simulink model "SWC_HALIN_CDD_type"  (R2021b)
settings: Solver=FixedStepDiscrete  StartTime=0.0  StopTime=10.0  FixedStep=0.005  RelTol=1e-3
undefined symbols (not defined in the file or in its folder): C_TASK_5MS_S, DIDLen_APSFunConfig, DIDLen_AutoLock, DIDLen_AutoWipHSpdEN, DIDLen_DKCKey, DIDLen_DRLDis, DIDLen_DynoMode, DIDLen_FMHTimer, DIDLen_OBDReq, DIDLen_TestGroup, DIDLen_TireSize, DIDLen_TurnLampFLThreCurr, DIDLen_TurnLampFRThreCurr, DIDLen_TurnLampRLThreCurr, DIDLen_TurnLampRRThreCurr, DIDLen_USSConfig, DIDLen_WipRLSCmdCutFilter, DIDLen_WipRLSCmdHoldFilter, DIDLen_XWDMode, DIDNum_APSFunConfig, DIDNum_AutoLock, DIDNum_AutoWipHSpdEN, DIDNum_DKCKey, DIDNum_DRLDis, DIDNum_DynoMode, DIDNum_FMHTimer, DIDNum_OBDReq, DIDNum_TestGroup, DIDNum_TireSize, DIDNum_TurnLampFLThreCurr, DIDNum_TurnLampFRThreCurr, DIDNum_TurnLampRLThreCurr, DIDNum_TurnLampRRThreCurr, DIDNum_USSConfig, DIDNum_WipRLSCmdCutFilter, DIDNum_WipRLSCmdHoldFilter, DIDNum_XWDMode, ENUM_DRIVETRAIN_AWD, ENUM_DRIVETRAIN_FWD, ENUM_DRIVETRAIN_RWD, ENUM_REGENLEVEL_LV1, ENUM_REGENLEVEL_LV2, ENUM_REGENLEVEL_LV3, ENUM_REGENLEVEL_LV4, ENUM_REGENLEVEL_LV5, ENUM_REGENLEVEL_OPD, ENUM_TPMSSTA_FAT, ENUM_TPMSSTA_LOWBATTERY, ENUM_TPMSSTA_TRIGGER, FALSE, FIVE_INT, FOUR_INT, KHAL_CANBusOffDebounce_s, KHAL_DefaultRegenMode_enum, KHAL_DKCDecryptEnable_flg_ovrdflg, KHAL_DKCDecryptEnable_flg_ovrdval, KHAL_RandomNumberY1_enum, KHAL_RandomNumberY2_enum, KHAL_RandomNumberY_ovrdflg, KHAL_TPMSRESBUTT_flg_ovrdflg ... (+9)
libraries: simulink x229, FVT_lib x29, hcu_lib x25, hdlsllib x15
(part 1 of 8)
settings Model: DataDictionary=APPTypes.sldd  Creator=FVT23010  LastModifiedBy=FVT23010
settings DataIOCC: SaveFormat=StructureWithTime
settings OptimizationCC: DefaultParameterBehavior=Inlined  EnhancedBackFolding=on  PassReuseOutputArgsAs=Individual arguments  ZeroExternalMemoryAtStartup=off  ZeroInternalMemoryAtStartup=off  OptimizeBlockOrder=speed  DifferentSizesBufferReuse=on  OptimizationCustomize=off  EfficientTunableParamExpr=on
settings DebuggingCC: ParameterTunabilityLossMsg=error
settings ModelReferenceCC: ModelReferenceNumInstancesAllowed=Single
settings SFSimCC: MATLABDynamicMemAlloc=off
settings RTWCC: Description=AUTOSAR  SystemTargetFile=autosar.tlc  GenCodeOnly=on  TemplateMakefile=ert_default_tmf
settings CodeAppCC: ForceParamTrailComments=on  IgnoreCustomStorageClasses=off  OperatorAnnotations=on  SimulinkDataObjDesc=on  SFDataObjDesc=on  InsertBlockDesc=on
settings STFCustomTargetCC: TargetLangStandard=C99 (ISO)  MultiwordLength=256  ParMdlRefBuildCompliant=on  CompOptLevelCompliant=on  IncludeMdlTerminateFcn=off  CombineOutputUpdateFcns=on  SuppressErrorStatus=on  ERTCustomFileBanners=on  SupportNonFinite=off  SupportComplex=off  SupportContinuousTime=off  SupportNonInlinedSFcns=off  RemoveResetFunc=on  MATLABClassNameForMDSCustomization=Simulink.SoftwareTarget.ERTCustomization  AutosarCompliant=on  GRTInterface=off  UseToolchainInfoCompliant=on  LookupTableObjectStructAxisOrder=2,1,3,4,...  LUTObjectStructOrderEvenSpacing=Size,Table,Breakpoints  SystemTargetFile=autosar.tlc
settings ERTTargetCC: TargetLangStandard=C99 (ISO)  ConcurrentExecutionCompliant=off  IncludeMdlTerminateFcn=off  SuppressErrorStatus=on  SupportNonFinite=off  SupportComplex=off  ModelStepFunctionPrototypeControlCompliant=off  CPPClassGenCompliant=off  AutosarCompliant=on  LookupTableObjectStructAxisOrder=2,1,3,4,...  LUTObjectStructOrderEvenSpacing=Size,Table,Breakpoints  InlinedParameterPlacement=NonHierarchical  ERTCustomFileTemplate=example_file_process.tlc

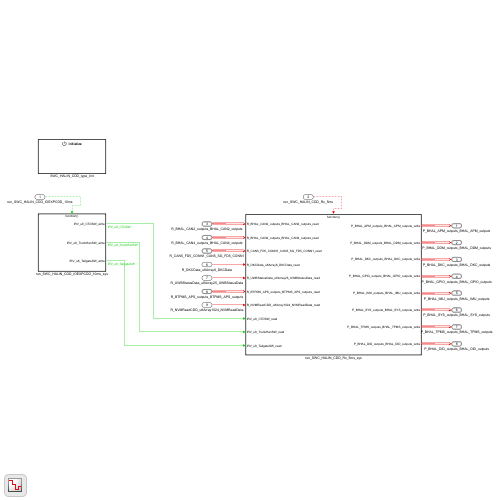
[thumbnail: Simulink's stored preview of the top-level diagram]
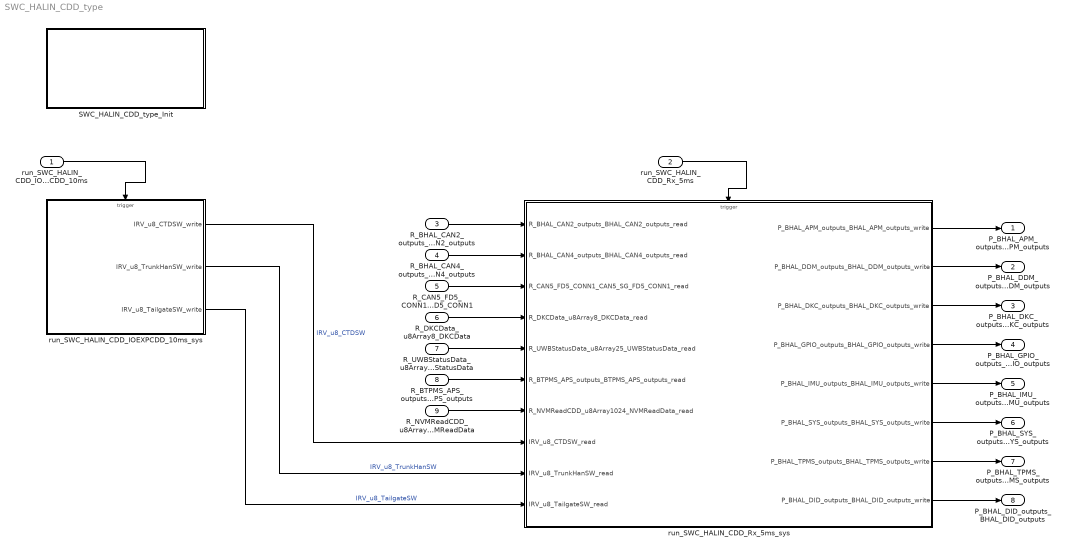
== system SWC_HALIN_CDD_type ==
  run_SWC_HALIN_CDD_IOEXPCDD_10ms : Inport  SampleTime=0.01  OutputFunctionCall=on
  run_SWC_HALIN_CDD_Rx_5ms : Inport  Port=2  SampleTime=0.005  OutputFunctionCall=on
  R_BHAL_CAN2_outputs_BHAL_CAN2_outputs : Inport  Port=3  OutDataTypeStr=Bus: BHAL_CAN2_outputs  PortDimensions=1  BusOutputAsStruct=on
  R_BHAL_CAN4_outputs_BHAL_CAN4_outputs : Inport  Port=4  OutDataTypeStr=Bus: BHAL_CAN4_outputs  PortDimensions=1  BusOutputAsStruct=on
  R_CAN5_FD5_CONN1_CAN5_SG_FD5_CONN1 : Inport  Port=5  OutDataTypeStr=Bus: DT_CAN5_SG_FD5_CONN1  PortDimensions=1  BusOutputAsStruct=on
  R_DKCData_u8Array8_DKCData : Inport  Port=6  OutDataTypeStr=uint8  PortDimensions=8
  R_UWBStatusData_u8Array25_UWBStatusData : Inport  Port=7  OutDataTypeStr=uint8  PortDimensions=25
  R_BTPMS_APS_outputs_BTPMS_APS_outputs : Inport  Port=8  OutDataTypeStr=Bus: DT_TPMS_APS_outputs  PortDimensions=1  BusOutputAsStruct=on
  R_NVMReadCDD_u8Array1024_NVMReadData : Inport  Port=9  OutDataTypeStr=uint8  PortDimensions=1024
  SWC_HALIN_CDD_type_Init : Subsystem
  run_SWC_HALIN_CDD_IOEXPCDD_10ms_sys : Subsystem
  run_SWC_HALIN_CDD_Rx_5ms_sys : Subsystem
  P_BHAL_APM_outputs_BHAL_APM_outputs : Outport  OutDataTypeStr=Bus: BHAL_APM_outputs  PortDimensions=1  BusOutputAsStruct=on
  P_BHAL_DDM_outputs_BHAL_DDM_outputs : Outport  Port=2  OutDataTypeStr=Bus: BHAL_DDM_outputs  PortDimensions=1  BusOutputAsStruct=on
  P_BHAL_DKC_outputs_BHAL_DKC_outputs : Outport  Port=3  OutDataTypeStr=Bus: BHAL_DKC_outputs  PortDimensions=1  BusOutputAsStruct=on
  P_BHAL_GPIO_outputs_BHAL_GPIO_outputs : Outport  Port=4  OutDataTypeStr=Bus: BHAL_GPIO_outputs  PortDimensions=1  BusOutputAsStruct=on
  P_BHAL_IMU_outputs_BHAL_IMU_outputs : Outport  Port=5  OutDataTypeStr=Bus: BHAL_IMU_outputs  PortDimensions=1  BusOutputAsStruct=on
  P_BHAL_SYS_outputs_BHAL_SYS_outputs : Outport  Port=6  OutDataTypeStr=Bus: BHAL_SYS_outputs  PortDimensions=1  BusOutputAsStruct=on
  P_BHAL_TPMS_outputs_BHAL_TPMS_outputs : Outport  Port=7  OutDataTypeStr=Bus: BHAL_TPMS_outputs  PortDimensions=1  BusOutputAsStruct=on
  P_BHAL_DID_outputs_BHAL_DID_outputs : Outport  Port=8  OutDataTypeStr=Bus: BHAL_DID_outputs  PortDimensions=1  BusOutputAsStruct=on
  wires:
  R_BHAL_CAN2_outputs_BHAL_CAN2_outputs/1 -> run_SWC_HALIN_CDD_Rx_5ms_sys/1(R_BHAL_CAN2_outputs_BHAL_CAN2_outputs_read)
  R_BHAL_CAN4_outputs_BHAL_CAN4_outputs/1 -> run_SWC_HALIN_CDD_Rx_5ms_sys/2(R_BHAL_CAN4_outputs_BHAL_CAN4_outputs_read)
  R_CAN5_FD5_CONN1_CAN5_SG_FD5_CONN1/1 -> run_SWC_HALIN_CDD_Rx_5ms_sys/3(R_CAN5_FD5_CONN1_CAN5_SG_FD5_CONN1_read)
  R_DKCData_u8Array8_DKCData/1 -> run_SWC_HALIN_CDD_Rx_5ms_sys/4(R_DKCData_u8Array8_DKCData_read)
  R_UWBStatusData_u8Array25_UWBStatusData/1 -> run_SWC_HALIN_CDD_Rx_5ms_sys/5(R_UWBStatusData_u8Array25_UWBStatusData_read)
  R_BTPMS_APS_outputs_BTPMS_APS_outputs/1 -> run_SWC_HALIN_CDD_Rx_5ms_sys/6(R_BTPMS_APS_outputs_BTPMS_APS_outputs_read)
  R_NVMReadCDD_u8Array1024_NVMReadData/1 -> run_SWC_HALIN_CDD_Rx_5ms_sys/7(R_NVMReadCDD_u8Array1024_NVMReadData_read)
  run_SWC_HALIN_CDD_Rx_5ms_sys/1(P_BHAL_APM_outputs_BHAL_APM_outputs_write) -> P_BHAL_APM_outputs_BHAL_APM_outputs/1
  run_SWC_HALIN_CDD_Rx_5ms_sys/2(P_BHAL_DDM_outputs_BHAL_DDM_outputs_write) -> P_BHAL_DDM_outputs_BHAL_DDM_outputs/1
  run_SWC_HALIN_CDD_Rx_5ms_sys/3(P_BHAL_DKC_outputs_BHAL_DKC_outputs_write) -> P_BHAL_DKC_outputs_BHAL_DKC_outputs/1
  run_SWC_HALIN_CDD_Rx_5ms_sys/4(P_BHAL_GPIO_outputs_BHAL_GPIO_outputs_write) -> P_BHAL_GPIO_outputs_BHAL_GPIO_outputs/1
  run_SWC_HALIN_CDD_Rx_5ms_sys/5(P_BHAL_IMU_outputs_BHAL_IMU_outputs_write) -> P_BHAL_IMU_outputs_BHAL_IMU_outputs/1
  run_SWC_HALIN_CDD_Rx_5ms_sys/6(P_BHAL_SYS_outputs_BHAL_SYS_outputs_write) -> P_BHAL_SYS_outputs_BHAL_SYS_outputs/1
  run_SWC_HALIN_CDD_Rx_5ms_sys/7(P_BHAL_TPMS_outputs_BHAL_TPMS_outputs_write) -> P_BHAL_TPMS_outputs_BHAL_TPMS_outputs/1
  run_SWC_HALIN_CDD_Rx_5ms_sys/8(P_BHAL_DID_outputs_BHAL_DID_outputs_write) -> P_BHAL_DID_outputs_BHAL_DID_outputs/1
  run_SWC_HALIN_CDD_IOEXPCDD_10ms_sys/1(IRV_u8_CTDSW_write) -> run_SWC_HALIN_CDD_Rx_5ms_sys/8(IRV_u8_CTDSW_read)  "IRV_u8_CTDSW"
  run_SWC_HALIN_CDD_IOEXPCDD_10ms_sys/2(IRV_u8_TrunkHanSW_write) -> run_SWC_HALIN_CDD_Rx_5ms_sys/9(IRV_u8_TrunkHanSW_read)  "IRV_u8_TrunkHanSW"
  run_SWC_HALIN_CDD_IOEXPCDD_10ms_sys/3(IRV_u8_TailgateSW_write) -> run_SWC_HALIN_CDD_Rx_5ms_sys/10(IRV_u8_TailgateSW_read)  "IRV_u8_TailgateSW"
  run_SWC_HALIN_CDD_IOEXPCDD_10ms/1 -> run_SWC_HALIN_CDD_IOEXPCDD_10ms_sys/Trigger
  run_SWC_HALIN_CDD_Rx_5ms/1 -> run_SWC_HALIN_CDD_Rx_5ms_sys/Trigger

== system SWC_HALIN_CDD_type/SWC_HALIN_CDD_type_Init ==
  Event Listener : EventListener  EventName=reset

== system SWC_HALIN_CDD_type/run_SWC_HALIN_CDD_IOEXPCDD_10ms_sys ==
  function : TriggerPort  TriggerType=function-call  VariantControl=(inherit)  SampleTimeType=periodic  SampleTime=-1
  R_IOExpIN_CDD_CSOP_IOExpGetVal : FunctionCaller  FunctionPrototype=[u8_CTDSW,u8_TrunkHanSW,u8_TailgateSW] = R_IOExpIN_CDD_CSOP_IOExpGetVal()  OutputArgumentSpecifications=uint8(1), uint8(1), uint8(1)
  IRV_u8_CTDSW_write : Outport  OutDataTypeStr=uint8  PortDimensions=1
  IRV_u8_TrunkHanSW_write : Outport  Port=2  OutDataTypeStr=uint8  PortDimensions=1
  IRV_u8_TailgateSW_write : Outport  Port=3  OutDataTypeStr=uint8  PortDimensions=1
  wires:
  R_IOExpIN_CDD_CSOP_IOExpGetVal/1 -> IRV_u8_CTDSW_write/1
  R_IOExpIN_CDD_CSOP_IOExpGetVal/2 -> IRV_u8_TrunkHanSW_write/1
  R_IOExpIN_CDD_CSOP_IOExpGetVal/3 -> IRV_u8_TailgateSW_write/1

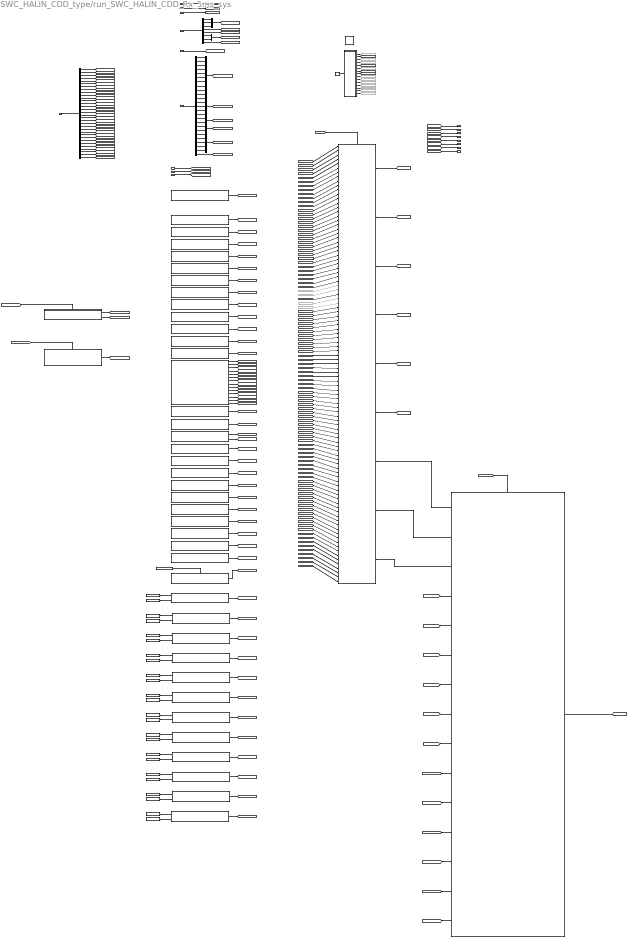
== system SWC_HALIN_CDD_type/run_SWC_HALIN_CDD_Rx_5ms_sys ==
  R_BHAL_CAN2_outputs_BHAL_CAN2_outputs_read : Inport
  R_BHAL_CAN4_outputs_BHAL_CAN4_outputs_read : Inport  Port=2
  R_CAN5_FD5_CONN1_CAN5_SG_FD5_CONN1_read : Inport  Port=3
  R_DKCData_u8Array8_DKCData_read : Inport  Port=4
  R_UWBStatusData_u8Array25_UWBStatusData_read : Inport  Port=5
  R_BTPMS_APS_outputs_BTPMS_APS_outputs_read : Inport  Port=6
  R_NVMReadCDD_u8Array1024_NVMReadData_read : Inport  Port=7
  IRV_u8_CTDSW_read : Inport  Port=8
  IRV_u8_TrunkHanSW_read : Inport  Port=9
  IRV_u8_TailgateSW_read : Inport  Port=10
  function : TriggerPort  TriggerType=function-call  VariantControl=(inherit)  SampleTimeType=periodic  SampleTime=-1
  Bus Selector : BusSelector  OutputSignals=u16Array4_ApsInDist,u8Array12_ApsInUssSta,u8Array8_ApsInLevel,u8Array8_PasInDist,u8Array9_TPMSData,u8_ApsInPASChime,u8_ApsInSensorLayout,u8_ApsInSysFailSta,u8_ApsInSysMode,u8_TPMSDataInSta,u8_GetAPS_Progress_PCT,u8_GetAPS_RQ_Display,u8_GetAPS_SW_Ver,u8_GetAPS_HW_Ver,u8_GetAPS_ExitCondition,f32_GetAPS_Angle_Target,u8_GetAPS_Sta_System,u8_GetAPS_V_Rq_EPAS_Ctrl,u8_GetAPS_Rq_EPAS_Ctrl,u8_GetAPS_Req,f32_GetAPS_DecReq,u8_GetAPS_DecReq_A,f32_GetAPS_SpeedCmd,u8_GetAPS_ShftPosnReq,u8_GetAPS_VMC_Req_A,u8_GetCAAS_Sta,u8_GetCAAS_VMC_Req_A,u8_GetAPS_PwrReq_cmd,u8_GetRAPS_BCM_LockReq_Cmd,u8_GetRAPS_BCM_Lamp_Cmd,u8_GetRAPS_ErrWarn_Sta,u8_GetRAPS_ErrLv1_flg
  Constant{10,16..17,21,25,29} (6 alike) : Constant  Value=ZERO_INT
  Constant{6,9,11..13,20,24,28,32} (9 alike) : Constant  Value=ONE_INT
  Constant14 : Constant  Value=TWO_INT
  Constant15 : Constant  Value=TWO_INT
  Constant18 : Constant  Value=THREE_INT
  Constant19 : Constant  Value=THREE_INT
  Constant22 : Constant  Value=FOUR_INT
  Constant23 : Constant  Value=FOUR_INT
  Constant26 : Constant  Value=FIVE_INT
  Constant27 : Constant  Value=FIVE_INT
  Constant30 : Constant  Value=SIX_INT
  Constant31 : Constant  Value=SIX_INT
  Constant5 : Constant  Value=FALSE
  Constant8 : Constant  Value=KINP_ReadVinCode_flg
  DIDGet_Subsystem : Subsystem
  Demux : Demux  Outputs=8
  Demux1 : Demux  Outputs=25
  From91 : From  Commented=on  GotoTag=u8_DidStaXWD
  From92 : From  Commented=on  GotoTag=u8Array8_DidDataDKC
  From96 : From  Commented=on  GotoTag=u8_DidDataXWD
  From97 : From  Commented=on  GotoTag=u8_DidStaDKC
  Goto100 : Goto  Commented=on  GotoTag=trig_Read_NVM_00
  Goto101 : Goto  Commented=on  GotoTag=trig_HAL_OUTAFTER_50_1
  Goto106 : Goto  Commented=on  GotoTag=trig_GetNMID
  Goto119 : Goto  Commented=on  GotoTag=trig_HAL_DKC_10_3
  Goto91 : Goto  Commented=on  GotoTag=trig_WDG
  Goto94 : Goto  Commented=on  GotoTag=trig_HAL_OUT_50
  Goto95 : Goto  Commented=on  GotoTag=trig_OUTP_AFTER_40_1
  Goto96 : Goto  Commented=on  GotoTag=trig_OUTP_40
  Goto97 : Goto  Commented=on  GotoTag=trig_APP_30
  Goto98 : Goto  Commented=on  GotoTag=trig_INP_20
  Goto99 : Goto  Commented=on  GotoTag=trig_HAL_IN_10
  Halin_CDD : Subsystem
      settings: RTWSystemCode=Nonreusable function  RTWFcnNameOpts=Use subsystem name  RTWFileNameOpts=Use subsystem name
  Mux : Mux  Inputs=3
  Mux1 : Mux  Inputs=2
  Mux2 : Mux  Inputs=10
  Mux3 : Mux  Inputs=5
  Mux4 : Mux  Inputs=2
  Mux5 : Mux  Inputs=2
  Mux6 : Mux  Inputs=5
  R_HALINCDD_CSOP_AnyNmID : FunctionCaller  FunctionPrototype=u8_AnyNMID = R_HALINCDD_CSOP_AnyNmID()  OutputArgumentSpecifications=uint8(1)
  R_HALINCDD_CSOP_CAN1BusOff : FunctionCaller  FunctionPrototype=u8_CAN1BusOff = R_HALINCDD_CSOP_CAN1BusOff()  OutputArgumentSpecifications=uint8(1)
  R_HALINCDD_CSOP_CAN2BusOff : FunctionCaller  FunctionPrototype=u8_CAN2BusOff = R_HALINCDD_CSOP_CAN2BusOff()  OutputArgumentSpecifications=uint8(1)
  R_HALINCDD_CSOP_CAN3BusOff : FunctionCaller  FunctionPrototype=u8_CAN3BusOff = R_HALINCDD_CSOP_CAN3BusOff()  OutputArgumentSpecifications=uint8(1)
  R_HALINCDD_CSOP_CAN4BusOff : FunctionCaller  FunctionPrototype=u8_CAN4BusOff = R_HALINCDD_CSOP_CAN4BusOff()  OutputArgumentSpecifications=uint8(1)
  R_HALINCDD_CSOP_CAN5BusOff : FunctionCaller  FunctionPrototype=u8_CAN5BusOff = R_HALINCDD_CSOP_CAN5BusOff()  OutputArgumentSpecifications=uint8(1)
  R_HALINCDD_CSOP_CAN6BusOff : FunctionCaller  FunctionPrototype=u8_CAN6BusOff = R_HALINCDD_CSOP_CAN6BusOff()  OutputArgumentSpecifications=uint8(1)
  R_HALINCDD_CSOP_GetAcoreReadyToSleep : FunctionCaller  FunctionPrototype=s8_AcoreReadyToSleep = R_HALINCDD_CSOP_GetAcoreReadyToSleep()  OutputArgumentSpecifications=int8(1)
  R_HALINCDD_CSOP_GetAcoreRebootCmd : FunctionCaller  FunctionPrototype=u8_AcoreRebootCmd = R_HALINCDD_CSOP_GetAcoreRebootCmd()  OutputArgumentSpecifications=uint8(1)
  R_HALINCDD_CSOP_GetAuxBattVoltage : FunctionCaller  FunctionPrototype=u16_AuxBattVol100mV = R_HALINCDD_CSOP_GetAuxBattVoltage()  OutputArgumentSpecifications=uint16(1)
  R_HALINCDD_CSOP_GetBootPath : FunctionCaller  FunctionPrototype=u32_BootPath = R_HALINCDD_CSOP_GetBootPath()  OutputArgumentSpecifications=uint32(1)
  R_HALINCDD_CSOP_GetBootReason : FunctionCaller  FunctionPrototype=u8_BootReason = R_HALINCDD_CSOP_GetBootReason()  OutputArgumentSpecifications=uint8(1)
  R_HALINCDD_CSOP_GetEvccAplusPwrUpReq : FunctionCaller  FunctionPrototype=u8_EvccAplusPwrUpReq = R_HALINCDD_CSOP_GetEvccAplusPwrUpReq()  OutputArgumentSpecifications=uint8(1)
  R_HALINCDD_CSOP_GetNmState : FunctionCaller  FunctionPrototype=u8_CurrentNMState = R_HALINCDD_CSOP_GetNmState()  OutputArgumentSpecifications=uint8(1)
  R_HALINCDD_CSOP_GetNvmProtectState : FunctionCaller  FunctionPrototype=u8_NvmProtectSta = R_HALINCDD_CSOP_GetNvmProtectState()  OutputArgumentSpecifications=uint8(1)
  R_HALINCDD_CSOP_GetSWID : FunctionCaller  FunctionPrototype=u8Array33_SWID = R_HALINCDD_CSOP_GetSWID()  OutputArgumentSpecifications=uint8([1;1;1;1;1;1;1;1;1;1;1;1;1;1;1;1;1;1;1;1;1;1;1;1;1;1;1;1;1;1;1;1;1])
  R_HALINCDD_CSOP_GetVinCode : Subsystem
  R_HALINCDD_CSOP_GetVinpAllowMoveThdOta : FunctionCaller  FunctionPrototype=u8_AllowMovThdOTA = R_HALINCDD_CSOP_GetVinpAllowMoveThdOta()  OutputArgumentSpecifications=uint8(1)
  R_HALINCDD_CSOP_GetVinpPwrReqOta : FunctionCaller  FunctionPrototype=u8_PwrReqOTA = R_HALINCDD_CSOP_GetVinpPwrReqOta()  OutputArgumentSpecifications=uint8(1)
  R_HALINCDD_CSOP_GetWISR : FunctionCaller  FunctionPrototype=u32_WISR = R_HALINCDD_CSOP_GetWISR()  OutputArgumentSpecifications=uint32(1)
  R_HALINCDD_CSOP_HALINCDD_DIRECT : FunctionCaller  FunctionPrototype=[u8_BrakeSW,u8_BrakeLamp,f32_Pedal1Vol,f32_Pedal2Vol,f32_Pedal1Ref5V,f32_Pedal2Ref5V,u8_DrDoorSW,u8_PsDoorSW,u8_RRDoorSW,u8_RLDoorSW,u8_HoodSW,u8_HazardSW,u8_SeatSW,u8_CrashSignal] = R_HALINCDD_CSOP_HALINCDD_DIRECT()  OutputArgumentSpecifications=uint8(1), uint8(1), single(1), single(1), single(1), single(1), uint8(1), uint8(1), uint8(1), uint8(1), uint8(1), uint8(1), uint8(1), uint8(1)
  R_HALINCDD_CSOP_ReadPedalZeroPosReq : FunctionCaller  FunctionPrototype=u8_ReadPedalZeroPosReq = R_HALINCDD_CSOP_ReadPedalZeroPosReq()  OutputArgumentSpecifications=uint8(1)
  R_HALINCDD_CSOP_ResetPedalZeroPosReq : FunctionCaller  FunctionPrototype=u8_ResetPedalZeroPosReq = R_HALINCDD_CSOP_ResetPedalZeroPosReq()  OutputArgumentSpecifications=uint8(1)
  R_HALINCDD_CSOP_TPMSSensorIDRegGetSta : FunctionCaller  FunctionPrototype=u8_TPMSSensorIDRegSta = R_HALINCDD_CSOP_TPMSSensorIDRegGetSta()  OutputArgumentSpecifications=uint8(1)
  R_HALINCDD_CSOP_nmGetCan1RxErrorCount : FunctionCaller  FunctionPrototype=u8_pCan1RxErrorCount = R_HALINCDD_CSOP_nmGetCan1RxErrorCount(u8_canChannel,u8_isGetRx)  InputArgumentSpecifications=uint8(1), uint8(1)  OutputArgumentSpecifications=uint8(1)
  R_HALINCDD_CSOP_nmGetCan1TxErrorCount : FunctionCaller  FunctionPrototype=u8_pCan1TxErrorCount = R_HALINCDD_CSOP_nmGetCan1TxErrorCount(u8_canChannel,u8_isGetRx)  InputArgumentSpecifications=uint8(1), uint8(1)  OutputArgumentSpecifications=uint8(1)
  R_HALINCDD_CSOP_nmGetCan2RxErrorCount : FunctionCaller  FunctionPrototype=u8_pCan2RxErrorCount = R_HALINCDD_CSOP_nmGetCan2RxErrorCount(u8_canChannel,u8_isGetRx)  InputArgumentSpecifications=uint8(1), uint8(1)  OutputArgumentSpecifications=uint8(1)
  R_HALINCDD_CSOP_nmGetCan2TxErrorCount : FunctionCaller  FunctionPrototype=u8_pCan2TxErrorCount = R_HALINCDD_CSOP_nmGetCan2TxErrorCount(u8_canChannel,u8_isGetRx)  InputArgumentSpecifications=uint8(1), uint8(1)  OutputArgumentSpecifications=uint8(1)
  R_HALINCDD_CSOP_nmGetCan3RxErrorCount : FunctionCaller  FunctionPrototype=u8_pCan3RxErrorCount = R_HALINCDD_CSOP_nmGetCan3RxErrorCount(u8_canChannel,u8_isGetRx)  InputArgumentSpecifications=uint8(1), uint8(1)  OutputArgumentSpecifications=uint8(1)
  R_HALINCDD_CSOP_nmGetCan3TxErrorCount : FunctionCaller  FunctionPrototype=u8_pCan3TxErrorCount = R_HALINCDD_CSOP_nmGetCan3TxErrorCount(u8_canChannel,u8_isGetRx)  InputArgumentSpecifications=uint8(1), uint8(1)  OutputArgumentSpecifications=uint8(1)
  R_HALINCDD_CSOP_nmGetCan4RxErrorCount : FunctionCaller  FunctionPrototype=u8_pCan4RxErrorCount = R_HALINCDD_CSOP_nmGetCan4RxErrorCount(u8_canChannel,u8_isGetRx)  InputArgumentSpecifications=uint8(1), uint8(1)  OutputArgumentSpecifications=uint8(1)
  R_HALINCDD_CSOP_nmGetCan4TxErrorCount : FunctionCaller  FunctionPrototype=u8_pCan4TxErrorCount = R_HALINCDD_CSOP_nmGetCan4TxErrorCount(u8_canChannel,u8_isGetRx)  InputArgumentSpecifications=uint8(1), uint8(1)  OutputArgumentSpecifications=uint8(1)
  R_HALINCDD_CSOP_nmGetCan5RxErrorCount : FunctionCaller  FunctionPrototype=u8_pCan5RxErrorCount = R_HALINCDD_CSOP_nmGetCan5RxErrorCount(u8_canChannel,u8_isGetRx)  InputArgumentSpecifications=uint8(1), uint8(1)  OutputArgumentSpecifications=uint8(1)
  R_HALINCDD_CSOP_nmGetCan5TxErrorCount : FunctionCaller  FunctionPrototype=u8_pCan5TxErrorCount = R_HALINCDD_CSOP_nmGetCan5TxErrorCount(u8_canChannel,u8_isGetRx)  InputArgumentSpecifications=uint8(1), uint8(1)  OutputArgumentSpecifications=uint8(1)
  R_HALINCDD_CSOP_nmGetCan6RxErrorCount : FunctionCaller  FunctionPrototype=u8_pCan6RxErrorCount = R_HALINCDD_CSOP_nmGetCan6RxErrorCount(u8_canChannel,u8_isGetRx)  InputArgumentSpecifications=uint8(1), uint8(1)  OutputArgumentSpecifications=uint8(1)
  R_HALINCDD_CSOP_nmGetCan6TxErrorCount : FunctionCaller  FunctionPrototype=u8_pCan6TxErrorCount = R_HALINCDD_CSOP_nmGetCan6TxErrorCount(u8_canChannel,u8_isGetRx)  InputArgumentSpecifications=uint8(1), uint8(1)  OutputArgumentSpecifications=uint8(1)
  R_HALINCDD_u8Array4_HWID : FunctionCaller  FunctionPrototype=u8Array4_HWID = R_HALINCDD_u8Array4_HWID()  OutputArgumentSpecifications=uint8([1;1;1;1])
  R_HALIN_IMU_CSOP_IMUGetOffsetVal : Subsystem
  R_HALIN_IMU_CSOP_IMUGetSixAxisVal : FunctionCaller  FunctionPrototype=[s16_IMUSixAxisVal,u8_IMUSixAxisValSta] = R_HALIN_IMU_CSOP_IMUGetSixAxisVal()  OutputArgumentSpecifications=int16([1;1;1;1;1;1]), uint8(1)
  R_UDSCDD_CSOP_DdmClearDTCNotification : FunctionCaller  FunctionPrototype=u8_ClearDTCcmd = R_UDSCDD_CSOP_DdmClearDTCNotification()  OutputArgumentSpecifications=uint8(1)
  R_UDSCDD_CSOP_DdmClearZevDTCNotification : FunctionCaller  FunctionPrototype=u8_ClearZevDTCcmd = R_UDSCDD_CSOP_DdmClearZevDTCNotification()  OutputArgumentSpecifications=uint8(1)
  Subsystem : Subsystem
  hcu_main_sched : Stateflow chart  TreatAsAtomicUnit=on
  P_BHAL_APM_outputs_BHAL_APM_outputs_write : Outport
  P_BHAL_DDM_outputs_BHAL_DDM_outputs_write : Outport  Port=2
  P_BHAL_DKC_outputs_BHAL_DKC_outputs_write : Outport  Port=3
  P_BHAL_GPIO_outputs_BHAL_GPIO_outputs_write : Outport  Port=4
  P_BHAL_IMU_outputs_BHAL_IMU_outputs_write : Outport  Port=5
  P_BHAL_SYS_outputs_BHAL_SYS_outputs_write : Outport  Port=6
  P_BHAL_TPMS_outputs_BHAL_TPMS_outputs_write : Outport  Port=7
  P_BHAL_DID_outputs_BHAL_DID_outputs_write : Outport  Port=8
  wires:
  IRV_u8_CTDSW_read/1 -> [u8_CTDSW]
  IRV_u8_TrunkHanSW_read/1 -> [u8_TrunkHanSW]
  IRV_u8_TailgateSW_read/1 -> [u8_TailgateSW]
  R_HALINCDD_CSOP_AnyNmID/1 -> [u8_AnyNMID]
  R_HALINCDD_CSOP_GetAcoreReadyToSleep/1 -> [s8_AcoreReadyToSleep]
  R_HALINCDD_CSOP_GetAuxBattVoltage/1 -> [u16_AuxBattVol100mV]
  R_HALINCDD_CSOP_GetBootReason/1 -> [u8_BootReason]
  R_HALINCDD_CSOP_GetBootPath/1 -> [u32_BootPath]
  R_HALINCDD_CSOP_GetEvccAplusPwrUpReq/1 -> [u8_EvccAplusPwrUpReq]
  R_HALINCDD_u8Array4_HWID/1 -> [u8Array4_HWID]
  R_HALINCDD_CSOP_GetNvmProtectState/1 -> [u8_NvmProtectSta]
  R_HALINCDD_CSOP_GetNmState/1 -> [u8_CurrentNMState]
  R_HALINCDD_CSOP_GetSWID/1 -> [u8Array33_SWID]
  R_HALINCDD_CSOP_GetVinpAllowMoveThdOta/1 -> [u8_AllowMovThdOTA]
  R_HALINCDD_CSOP_GetVinpPwrReqOta/1 -> [u8_PwrReqOTA]
  R_HALINCDD_CSOP_GetWISR/1 -> [u32_WISR]
  R_HALINCDD_CSOP_HALINCDD_DIRECT/1 -> [u8_BrakeSW]
  R_HALINCDD_CSOP_HALINCDD_DIRECT/2 -> [u8_BrakeLamp]
  R_HALINCDD_CSOP_HALINCDD_DIRECT/3 -> [f32_Pedal1Vol]
  R_HALINCDD_CSOP_HALINCDD_DIRECT/4 -> [f32_Pedal2Vol]
  R_HALINCDD_CSOP_HALINCDD_DIRECT/5 -> [f32_Pedal1Ref5V]
  R_HALINCDD_CSOP_HALINCDD_DIRECT/6 -> [f32_Pedal2Ref5V]
  R_HALINCDD_CSOP_HALINCDD_DIRECT/7 -> [u8_DrDoorSW]
  R_HALINCDD_CSOP_HALINCDD_DIRECT/8 -> [u8_PsDoorSW]
  R_HALINCDD_CSOP_HALINCDD_DIRECT/9 -> [u8_RRDoorSW]
  R_HALINCDD_CSOP_HALINCDD_DIRECT/10 -> [u8_RLDoorSW]
  R_HALINCDD_CSOP_HALINCDD_DIRECT/11 -> [u8_HoodSW]
  R_HALINCDD_CSOP_HALINCDD_DIRECT/12 -> [u8_HazardSW]
  R_HALINCDD_CSOP_HALINCDD_DIRECT/13 -> [u8_SeatSW]
  R_HALINCDD_CSOP_HALINCDD_DIRECT/14 -> [u8_CrashSignal]
  R_UDSCDD_CSOP_DdmClearDTCNotification/1 -> [u8_ClearDTCcmd]
  R_HALIN_IMU_CSOP_IMUGetSixAxisVal/1 -> [s16_IMUSixAxisVal]
  R_HALIN_IMU_CSOP_IMUGetSixAxisVal/2 -> [u8_IMUSixAxisValSta]
  R_HALINCDD_CSOP_GetAcoreRebootCmd/1 -> [u8_AcoreRebootCmd]
  R_HALINCDD_CSOP_CAN1BusOff/1 -> [u8_CAN1BusOff]
  R_HALINCDD_CSOP_CAN2BusOff/1 -> [u8_CAN2BusOff]
  R_HALINCDD_CSOP_CAN3BusOff/1 -> [u8_CAN3BusOff]
  R_HALINCDD_CSOP_CAN4BusOff/1 -> [u8_CAN4BusOff]
  R_HALINCDD_CSOP_CAN5BusOff/1 -> [u8_CAN5BusOff]
  R_HALINCDD_CSOP_CAN6BusOff/1 -> [u8_CAN6BusOff]
  R_HALINCDD_CSOP_TPMSSensorIDRegGetSta/1 -> [u8_TPMSSensorIDRegSta]
  R_HALINCDD_CSOP_ReadPedalZeroPosReq/1 -> [u8_ReadPedalZeroPosReq]
  R_HALINCDD_CSOP_ResetPedalZeroPosReq/1 -> [u8_ResetPedalZeroPosReq]
  R_HALINCDD_CSOP_GetVinCode/1(Out1) -> [u8Array17_VinCode]
  [trig_ReadIMUOffset_00] -> R_HALIN_IMU_CSOP_IMUGetOffsetVal/Trigger
  R_HALIN_IMU_CSOP_IMUGetOffsetVal/1(Out1) -> [s16_IMUOffsetVal]
  R_HALIN_IMU_CSOP_IMUGetOffsetVal/2(Out2) -> [u8_IMUOffsetValSta]
  [trig_GetDID] -> DIDGet_Subsystem/Trigger
  DIDGet_Subsystem/1(BHAL_DID_outputs) -> [BHAL_DID_outputs]
  R_UDSCDD_CSOP_DdmClearZevDTCNotification/1 -> [u8_ClearZevDTCcmd]
  hcu_main_sched/12(trig_OUTP_40()) -> Goto96/1
  hcu_main_sched/14(trig_HAL_OUT_50()) -> Goto94/1
  hcu_main_sched/8(trig_HAL_DKC_10_2()) -> [trig_HAL_DKC_10_2]
  hcu_main_sched/3(trig_WDG()) -> Goto91/1
  hcu_main_sched/9(trig_HAL_DKC_10_3()) -> Goto119/1
  hcu_main_sched/11(trig_APP_30()) -> Goto97/1
  hcu_main_sched/6(trig_HAL_IN_10()) -> Goto99/1
  hcu_main_sched/13(trig_OUTP_AFTER_40_1()) -> Goto95/1
  hcu_main_sched/1(trig_Read_NVM_00()) -> Goto100/1
  hcu_main_sched/4(trig_GetNMID()) -> Goto106/1
  hcu_main_sched/7(trig_HAL_CDD_10_1()) -> [trig_HAL_CDD_10_1]
  hcu_main_sched/2(trig_ReadIMUOffset_00()) -> [trig_ReadIMUOffset_00]
  hcu_main_sched/5(trig_GetDID()) -> [trig_GetDID]
  hcu_main_sched/10(trig_INP_20()) -> Goto98/1
  hcu_main_sched/15(trig_HAL_OUTAFTER_50_1()) -> Goto101/1
  Constant5/1 -> hcu_main_sched/1(VHAL_FusionSchedReq_flg)
  [BHAL_DID_outputs] -> P_BHAL_DID_outputs_BHAL_DID_outputs_write/1
  [BHAL_IMU_outputs] -> P_BHAL_IMU_outputs_BHAL_IMU_outputs_write/1
  [BHAL_SYS_outputs] -> P_BHAL_SYS_outputs_BHAL_SYS_outputs_write/1
  [BHAL_TPMS_outputs] -> P_BHAL_TPMS_outputs_BHAL_TPMS_outputs_write/1
  [BHAL_APM_outputs] -> P_BHAL_APM_outputs_BHAL_APM_outputs_write/1
  [BHAL_GPIO_outputs] -> P_BHAL_GPIO_outputs_BHAL_GPIO_outputs_write/1
  [BHAL_DKC_outputs] -> P_BHAL_DKC_outputs_BHAL_DKC_outputs_write/1
  [BHAL_DDM_outputs] -> P_BHAL_DDM_outputs_BHAL_DDM_outputs_write/1
  R_BHAL_CAN2_outputs_BHAL_CAN2_outputs_read/1 -> [BHAL_CAN2_outputs]
  R_BHAL_CAN4_outputs_BHAL_CAN4_outputs_read/1 -> [BHAL_CAN4_outputs]
  R_CAN5_FD5_CONN1_CAN5_SG_FD5_CONN1_read/1 -> [R_CAN5_FD5_CONN1]
  Mux/1 -> [u8Array3_DKCData]
  Demux/8 -> [s8_DKCUIDBLERSSI]
  Mux1/1 -> [u8Array2_DKCUIDBLEVol]
  Demux/2 -> Mux/2
  Demux/5 -> [u8_DKCUIDBLEStatus]
  R_NVMReadCDD_u8Array1024_NVMReadData_read/1 -> [u8Array1024_NvmReadArray]
  Demux/7 -> Mux1/2
  Demux/3 -> Mux/3
  R_DKCData_u8Array8_DKCData_read/1 -> Demux/1
  Demux/6 -> Mux1/1
  Demux/4 -> [u8_DKCButton]
  Demux/1 -> Mux/1
  Demux1/5 -> Mux2/5
  Demux1/6 -> Mux2/6
  Demux1/20 -> Mux6/1
  Mux2/1 -> [u8Array10_UWBDistanceCM]
  Mux6/1 -> [u8Array5_UWBRangingSta]
  Demux1/17 -> Mux4/2
  Demux1/25 -> [u8_UWBStaRangingONOFF]
  Mux5/1 -> [s8Array2_UWBpositionYCM]
  Demux1/23 -> Mux6/4
  Demux1/3 -> Mux2/3
  Demux1/14 -> Mux3/4
  Demux1/21 -> Mux6/2
  Demux1/15 -> Mux3/5
  Demux1/11 -> Mux3/1
  Demux1/8 -> Mux2/8
  Demux1/16 -> Mux4/1
  Mux4/1 -> [s8Array2_UWBpositionXCM]
  Demux1/1 -> Mux2/1
  Demux1/9 -> Mux2/9
  Demux1/7 -> Mux2/7
  Mux3/1 -> [s8Array5_UWBPowerdB]
  Demux1/22 -> Mux6/3
  R_UWBStatusData_u8Array25_UWBStatusData_read/1 -> Demux1/1
  Demux1/19 -> Mux5/2
  Demux1/18 -> Mux5/1
  Demux1/12 -> Mux3/2
  Demux1/10 -> Mux2/10
  Demux1/4 -> Mux2/4
  Demux1/24 -> Mux6/5
  Demux1/2 -> Mux2/2
  Demux1/13 -> Mux3/3
  [u8_CAN3BusOff] -> Halin_CDD/58(VHAL_CAN3BusOff_raw)
  Halin_CDD/2(BHAL_GPIO_outputs) -> [BHAL_GPIO_outputs]
  [u8_pCan2RxErrorCount] -> Halin_CDD/91(VHAL_CAN2RxErrorCount_raw)
  [u8Array9_TPMSData] -> Halin_CDD/39(TPMS_RawData)
  [u16_AuxBattVol100mV] -> Halin_CDD/48(VHAL_AuxBattVolmV_100mV)
  [u8_pCan1RxErrorCount] -> Halin_CDD/89(VHAL_CAN1RxErrorCount_raw)
  [u8_TrunkHanSW] -> Halin_CDD/21(VHAL_TrunkHanSW_flg)
  [u8_pCan5RxErrorCount] -> Halin_CDD/97(VHAL_CAN5RxErrorCount_raw)
  [trig_HAL_CDD_10_1] -> Halin_CDD/Trigger
  [u8_pCan2TxErrorCount] -> Halin_CDD/92(VHAL_CAN2TxErrorCount_raw)
  [s16_IMUOffsetVal] -> Halin_CDD/43(VHAL_IMUOffsetVal_raw)
  [u8_CTDSW] -> Halin_CDD/18(VHAL_CentralDoorLockSW_flg)
  Constant6/1 -> Halin_CDD/25(GetSWID_status)
  [u8_CAN5BusOff] -> Halin_CDD/60(VHAL_CAN5BusOff_raw)
  [u8_CAN4BusOff] -> Halin_CDD/59(VHAL_CAN4BusOff_raw)
  [u8_pCan1TxErrorCount] -> Halin_CDD/90(VHAL_CAN1TxErrorCount_raw)
  From96/1 -> Halin_CDD/34(VHAL_DidXWDData_enum)
  [u8_GetAPS_RQ_Display] -> Halin_CDD/63(u8_GetAPS_RQ_Display)
  [u8Array8_PasInDist] -> Halin_CDD/1(PASDistanceData)
  [u8_pCan5TxErrorCount] -> Halin_CDD/98(VHAL_CAN5TxErrorCount_raw)
  [u8_SeatSW] -> Halin_CDD/22(VHAL_SeatSW_flg)
  [u32_WISR] -> Halin_CDD/53(VHAL_WisrBootReason_raw32)
  [u8_CurrentNMState] -> Halin_CDD/28(VHAL_CurrentNmState_enum)
  [u8_pCan3RxErrorCount] -> Halin_CDD/93(VHAL_CAN3RxErrorCount_cnt)
  [u8_GetAPS_PwrReq_cmd] -> Halin_CDD/79(u8_GetAPS_PwrReq_cmd)
  [u8_BootReason] -> Halin_CDD/52(VHAL_PmicBootReason_enum)
  [u8_GetAPS_ShftPosnReq] -> Halin_CDD/75(u8_GetAPS_ShftPosnReq)
  [u8_IMUSixAxisValSta] -> Halin_CDD/46(VHAL_IMUSixAxisValSta_flg)
  [u8_GetAPS_V_Rq_EPAS_Ctrl] -> Halin_CDD/69(u8_GetAPS_V_Rq_EPAS_Ctrl)
  [BHAL_CAN2_outputs] -> Halin_CDD/40(BHAL_CAN2_outputs)
  [u8_GetRAPS_BCM_LockReq_Cmd] -> Halin_CDD/80(u8_GetRAPS_BCM_LockReq_Cmd)
  [u8_ApsInSensorLayout] -> Halin_CDD/6(SNSRLayoutIn)
  [u8_GetCAAS_VMC_Req_A] -> Halin_CDD/78(u8_GetCAAS_VMC_Req_A)
  [u8_GetAPS_DecReq_A] -> Halin_CDD/73(u8_GetAPS_DecReq_A)
  [f32_Pedal1Ref5V] -> Halin_CDD/49(VHAL_Pedal1Ref5V_raw)
  [s8_AcoreReadyToSleep] -> Halin_CDD/32(VHAL_AcoreReadyToSlp_flg)
  [u8_GetAPS_Sta_System] -> Halin_CDD/68(u8_GetAPS_Sta_System)
  [u8Array12_ApsInUssSta] -> Halin_CDD/4(APSFaultStaData)
  [u8_BrakeSW] -> Halin_CDD/11(VHAL_BrakeSWGPIO_flg)
  [f32_GetAPS_Angle_Target] -> Halin_CDD/67(f32_GetAPS_Angle_Target)
  [u32_BootPath] -> Halin_CDD/86(u32_BootPath)
  [u8_GetAPS_HW_Ver] -> Halin_CDD/65(u8_GetAPS_HW_Ver)
  [f32_GetAPS_DecReq] -> Halin_CDD/72(f32_GetAPS_DecReq)
  [u8_GetAPS_ExitCondition] -> Halin_CDD/66(u8_GetAPS_ExitCondition)
  Halin_CDD/3(BHAL_SYS_outputs) -> [BHAL_SYS_outputs]
  [u8_GetAPS_Req] -> Halin_CDD/71(u8_GetAPS_Req)
  [BHAL_CAN4_outputs] -> Halin_CDD/41(BHAL_CAN4_outputs)
  From91/1 -> Halin_CDD/33(VHAL_DidXWDSta_flg)
  [f32_GetAPS_SpeedCmd] -> Halin_CDD/74(f32_GetAPS_SpeedCmd)
  [u8_HoodSW] -> Halin_CDD/12(VHAL_HoodSW_flg)
  [u8_PsDoorSW] -> Halin_CDD/15(VHAL_PsDoorSW_flg)
  [u8_NvmProtectSta] -> Halin_CDD/47(VHAL_NvmProtectSta_flg)
  From97/1 -> Halin_CDD/36(VHAL_DIDVCUKeyReadSta_flg)
  [u8_EvccAplusPwrUpReq] -> Halin_CDD/31(VHAL_EvccAplusPwrUpReq_flg)
  [u8_CrashSignal] -> Halin_CDD/23(VHAL_CrashSignalGPIO_flg)
  Halin_CDD/4(BHAL_TPMS_outputs) -> [BHAL_TPMS_outputs]
  [u8_ResetPedalZeroPosReq] -> Halin_CDD/85(u8_ResetPedalZeroPosReq)
  [R_CAN5_FD5_CONN1] -> Halin_CDD/88(R_CAN5_FD5_CONN1)
  [VHAL_NetworkReqCalled_flg] -> Halin_CDD/51(VHAL_NetworkReqCalled_flg)
  [u16Array4_ApsInDist] -> Halin_CDD/2(APSDistanceData)
  [u8_AcoreRebootCmd] -> Halin_CDD/55(VHAL_AcoreRebootCmd_raw)
  [u8_GetAPS_Rq_EPAS_Ctrl] -> Halin_CDD/70(u8_GetAPS_Rq_EPAS_Ctrl)
  [u8Array33_SWID] -> Halin_CDD/26(GetSWID_data)
  [u8_AnyNMID] -> Halin_CDD/27(VHAL_AnyNMID_flg)
  Halin_CDD/5(BHAL_DDM_outputs) -> [BHAL_DDM_outputs]
  [u8Array4_HWID] -> Halin_CDD/24(u8_HWID_4byte)
  [u8_CAN6BusOff] -> Halin_CDD/61(VHAL_CAN6BusOff_raw)
  [u8Array8_ApsInLevel] -> Halin_CDD/3(APSLevelData)
  [u8_ApsInSysFailSta] -> Halin_CDD/7(StaFSyaIn)
  [u8_DrDoorSW] -> Halin_CDD/14(VHAL_DrDoorSW_flg)
  [u8_GetAPS_VMC_Req_A] -> Halin_CDD/76(u8_GetAPS_VMC_Req_A)
  [u8_RLDoorSW] -> Halin_CDD/17(VHAL_RLDoorSW_flg)
  [f32_Pedal2Ref5V] -> Halin_CDD/50(VHAL_Pedal2Ref5V_raw)
  [u8_CAN2BusOff] -> Halin_CDD/57(VHAL_CAN2BusOff_raw)
  [f32_Pedal2Vol] -> Halin_CDD/10(VHAL_AccelPedal2Vol_Raw)
  [u8_GetRAPS_BCM_Lamp_Cmd] -> Halin_CDD/81(u8_GetRAPS_BCM_Lamp_Cmd)
  [u8Array1024_NvmReadArray] -> Halin_CDD/35(HAL_NvmReadData_raw)
  [u8_BrakeLamp] -> Halin_CDD/20(VHAL_BrakeLampSW_flg)
  [u8_IMUOffsetValSta] -> Halin_CDD/45(VHAL_IMUOffsetValSta_flg)
  [u8_HazardSW] -> Halin_CDD/19(VHAL_HazardSW_flg)
  From92/1 -> Halin_CDD/37(VHAL_GetDIDVCUKey_enum)
  [u8_ApsInPASChime] -> Halin_CDD/5(ChimeIn)
  [s16_IMUSixAxisVal] -> Halin_CDD/44(VHAL_IMUSixAxisVal_raw)
  [u8_TPMSDataInSta] -> Halin_CDD/38(TPMS_DataIn_flg)
  [u8_pCan4TxErrorCount] -> Halin_CDD/96(VHAL_CAN4TxErrorCount_raw)
  [u8_pCan3TxErrorCount] -> Halin_CDD/94(VHAL_CAN3TxErrorCount_raw)
  [u8_pCan6TxErrorCount] -> Halin_CDD/100(VHAL_CAN6TxErrorCount_raw)
  [u8_RRDoorSW] -> Halin_CDD/16(VHAL_RRDoorSW_flg)
  [u8_ClearDTCcmd] -> Halin_CDD/42(VHAL_ClearDTCcmd_flg)
  [BHAL_DID_outputs] -> Halin_CDD/54(BHAL_DIDGetData_raw)
  [f32_Pedal1Vol] -> Halin_CDD/9(VHAL_AccelPedal1Vol_Raw)
  Halin_CDD/1(BHAL_APM_outputs) -> [BHAL_APM_outputs]
  [u8_ClearZevDTCcmd] -> Halin_CDD/101(VHAL_ClearZevDTCcmd_flg)
  [u8_GetRAPS_ErrLv1_flg] -> Halin_CDD/83(u8_GetRAPS_ErrLv1_flg)
  Halin_CDD/6(BHAL_IMU_outputs) -> [BHAL_IMU_outputs]
  [u8_GetAPS_Progress_PCT] -> Halin_CDD/62(u8_GetAPS_Progress_PCT)
  [u8_GetRAPS_ErrWarn_Sta] -> Halin_CDD/82(u8_GetRAPS_ErrWarn_Sta)
  [u8_CAN1BusOff] -> Halin_CDD/56(VHAL_CAN1BusOff_raw)
  [u8_TailgateSW] -> Halin_CDD/13(VHAL_TailgateSW_flg)
  [u8_pCan4RxErrorCount] -> Halin_CDD/95(VHAL_CAN4RxErrorCount_raw)
  [u8_AllowMovThdOTA] -> Halin_CDD/30(VHAL_AllowMovThd_OTA_enum)
  [u8_ApsInSysMode] -> Halin_CDD/8(ModOperationIn)
  [u8_GetAPS_SW_Ver] -> Halin_CDD/64(u8_GetAPS_SW_Ver)
  [u8_TPMSSensorIDRegSta] -> Halin_CDD/84(u8_TPMSSensorIDRegSta)
  [u8_PwrReqOTA] -> Halin_CDD/29(VHAL_PwrReq_OTA_enum)
  [u8_GetCAAS_Sta] -> Halin_CDD/77(u8_GetCAAS_Sta)
  [u8_pCan6RxErrorCount] -> Halin_CDD/99(VHAL_CAN6RxErrorCount_raw)
  [u8Array17_VinCode] -> Halin_CDD/87(u8Array17_VinCode)
  [u8_UWBStaRangingONOFF] -> Subsystem/15(u8_UWBStaRangingONOFF)
  [u8Array2_DKCUIDBLEVol] -> Subsystem/8(u8Array2_DKCUIDBLEVol)
  [s8Array5_UWBPowerdB] -> Subsystem/11(s8Array5_UWBPowerdB)
  [u8Array5_UWBRangingSta] -> Subsystem/14(u8Array5_UWBRangingSta)
  [u8_DKCUIDBLEStatus] -> Subsystem/7(u8_DKCUIDBLEStatus)
  [s8_DKCUIDBLERSSI] -> Subsystem/9(s8_DKCUIDBLERSSI)
  [u8Array10_UWBDistanceCM] -> Subsystem/10(u8Array10_UWBDistanceCM)
  [BHAL_CAN4_outputs] -> Subsystem/4(BHAL_CAN4_outputs)
  [u8Array3_DKCData] -> Subsystem/5(u8Array3_DKCData)
  [s8Array2_UWBpositionXCM] -> Subsystem/12(s8Array2_UWBpositionXCM)
  [s8Array2_UWBpositionYCM] -> Subsystem/13(s8Array2_UWBpositionYCM)
  [u8_DKCButton] -> Subsystem/6(u8_DKCButton)
  Halin_CDD/9(DKCRawData) -> Subsystem/3(DKCRawData)
  Halin_CDD/8(AESKey) -> Subsystem/2(AESKey)
  Halin_CDD/7(Enable_decrypt) -> Subsystem/1(Enable_Decrypt)
  [trig_HAL_DKC_10_2] -> Subsystem/Trigger
  Subsystem/1(BHAL_DKC_outputs) -> [BHAL_DKC_outputs]
  Constant8/1 -> R_HALINCDD_CSOP_GetVinCode/Enable
  Constant20/1 -> R_HALINCDD_CSOP_nmGetCan3RxErrorCount/2
  Constant14/1 -> R_HALINCDD_CSOP_nmGetCan2RxErrorCount/1
  Constant23/1 -> R_HALINCDD_CSOP_nmGetCan4TxErrorCount/1
  Constant25/1 -> R_HALINCDD_CSOP_nmGetCan5TxErrorCount/2
  Constant27/1 -> R_HALINCDD_CSOP_nmGetCan5TxErrorCount/1
  Constant32/1 -> R_HALINCDD_CSOP_nmGetCan6RxErrorCount/2
  Constant31/1 -> R_HALINCDD_CSOP_nmGetCan6TxErrorCount/1
  Constant30/1 -> R_HALINCDD_CSOP_nmGetCan6RxErrorCount/1
  Constant22/1 -> R_HALINCDD_CSOP_nmGetCan4RxErrorCount/1
  Constant18/1 -> R_HALINCDD_CSOP_nmGetCan3RxErrorCount/1
  Constant17/1 -> R_HALINCDD_CSOP_nmGetCan3TxErrorCount/2
  Constant15/1 -> R_HALINCDD_CSOP_nmGetCan2TxErrorCount/1
  Constant16/1 -> R_HALINCDD_CSOP_nmGetCan2TxErrorCount/2
  Constant12/1 -> R_HALINCDD_CSOP_nmGetCan1TxErrorCount/1
  Constant10/1 -> R_HALINCDD_CSOP_nmGetCan1TxErrorCount/2
  Constant24/1 -> R_HALINCDD_CSOP_nmGetCan4RxErrorCount/2
  Constant29/1 -> R_HALINCDD_CSOP_nmGetCan6TxErrorCount/2
  Constant21/1 -> R_HALINCDD_CSOP_nmGetCan4TxErrorCount/2
  Constant19/1 -> R_HALINCDD_CSOP_nmGetCan3TxErrorCount/1
  Constant13/1 -> R_HALINCDD_CSOP_nmGetCan2RxErrorCount/2
  Constant11/1 -> R_HALINCDD_CSOP_nmGetCan1RxErrorCount/1
  Constant9/1 -> R_HALINCDD_CSOP_nmGetCan1RxErrorCount/2
  Constant26/1 -> R_HALINCDD_CSOP_nmGetCan5RxErrorCount/1
  Constant28/1 -> R_HALINCDD_CSOP_nmGetCan5RxErrorCount/2
  R_HALINCDD_CSOP_nmGetCan6RxErrorCount/1 -> [u8_pCan6RxErrorCount]
  R_HALINCDD_CSOP_nmGetCan5RxErrorCount/1 -> [u8_pCan5RxErrorCount]
  R_HALINCDD_CSOP_nmGetCan4RxErrorCount/1 -> [u8_pCan4RxErrorCount]
  R_HALINCDD_CSOP_nmGetCan2TxErrorCount/1 -> [u8_pCan2TxErrorCount]
  R_HALINCDD_CSOP_nmGetCan5TxErrorCount/1 -> [u8_pCan5TxErrorCount]
  R_HALINCDD_CSOP_nmGetCan4TxErrorCount/1 -> [u8_pCan4TxErrorCount]
  R_HALINCDD_CSOP_nmGetCan1TxErrorCount/1 -> [u8_pCan1TxErrorCount]
  R_HALINCDD_CSOP_nmGetCan3TxErrorCount/1 -> [u8_pCan3TxErrorCount]
  R_HALINCDD_CSOP_nmGetCan1RxErrorCount/1 -> [u8_pCan1RxErrorCount]
  R_HALINCDD_CSOP_nmGetCan2RxErrorCount/1 -> [u8_pCan2RxErrorCount]
  R_HALINCDD_CSOP_nmGetCan6TxErrorCount/1 -> [u8_pCan6TxErrorCount]
  R_HALINCDD_CSOP_nmGetCan3RxErrorCount/1 -> [u8_pCan3RxErrorCount]
  Bus Selector/23 -> [f32_GetAPS_SpeedCmd]  "<f32_GetAPS_SpeedCmd>"
  Bus Selector/10 -> [u8_TPMSDataInSta]  "<u8_TPMSDataInSta>"
  Bus Selector/21 -> [f32_GetAPS_DecReq]  "<f32_GetAPS_DecReq>"
  Bus Selector/28 -> [u8_GetAPS_PwrReq_cmd]  "<u8_GetAPS_PwrReq_cmd>"
  Bus Selector/15 -> [u8_GetAPS_ExitCondition]  "<u8_GetAPS_ExitCondition>"
  Bus Selector/3 -> [u8Array8_ApsInLevel]  "<u8Array8_ApsInLevel>"
  Bus Selector/19 -> [u8_GetAPS_Rq_EPAS_Ctrl]  "<u8_GetAPS_Rq_EPAS_Ctrl>"
  Bus Selector/17 -> [u8_GetAPS_Sta_System]  "<u8_GetAPS_Sta_System>"
  Bus Selector/4 -> [u8Array8_PasInDist]  "<u8Array8_PasInDist>"
  Bus Selector/26 -> [u8_GetCAAS_Sta]  "<u8_GetCAAS_Sta>"
  Bus Selector/20 -> [u8_GetAPS_Req]  "<u8_GetAPS_Req>"
  Bus Selector/30 -> [u8_GetRAPS_BCM_Lamp_Cmd]  "<u8_GetRAPS_BCM_Lamp_Cmd>"
  Bus Selector/25 -> [u8_GetAPS_VMC_Req_A]  "<u8_GetAPS_VMC_Req_A>"
  Bus Selector/14 -> [u8_GetAPS_HW_Ver]  "<u8_GetAPS_HW_Ver>"
  Bus Selector/11 -> [u8_GetAPS_Progress_PCT]  "<u8_GetAPS_Progress_PCT>"
  Bus Selector/18 -> [u8_GetAPS_V_Rq_EPAS_Ctrl]  "<u8_GetAPS_V_Rq_EPAS_Ctrl>"
  Bus Selector/1 -> [u16Array4_ApsInDist]  "<u16Array4_ApsInDist>"
  Bus Selector/12 -> [u8_GetAPS_RQ_Display]  "<u8_GetAPS_RQ_Display>"
  Bus Selector/5 -> [u8Array9_TPMSData]  "<u8Array9_TPMSData>"
  Bus Selector/2 -> [u8Array12_ApsInUssSta]  "<u8Array12_ApsInUssSta>"
  Bus Selector/7 -> [u8_ApsInSensorLayout]  "<u8_ApsInSensorLayout>"
  Bus Selector/13 -> [u8_GetAPS_SW_Ver]  "<u8_GetAPS_SW_Ver>"
  Bus Selector/22 -> [u8_GetAPS_DecReq_A]  "<u8_GetAPS_DecReq_A>"
  Bus Selector/32 -> [u8_GetRAPS_ErrLv1_flg]  "<u8_GetRAPS_ErrLv1_flg>"
  Bus Selector/16 -> [f32_GetAPS_Angle_Target]  "<f32_GetAPS_Angle_Target>"
  Bus Selector/9 -> [u8_ApsInSysMode]  "<u8_ApsInSysMode>"
  Bus Selector/8 -> [u8_ApsInSysFailSta]  "<u8_ApsInSysFailSta>"
  Bus Selector/31 -> [u8_GetRAPS_ErrWarn_Sta]  "<u8_GetRAPS_ErrWarn_Sta>"
  Bus Selector/6 -> [u8_ApsInPASChime]  "<u8_ApsInPASChime>"
  Bus Selector/29 -> [u8_GetRAPS_BCM_LockReq_Cmd]  "<u8_GetRAPS_BCM_LockReq_Cmd>"
  Bus Selector/24 -> [u8_GetAPS_ShftPosnReq]  "<u8_GetAPS_ShftPosnReq>"
  Bus Selector/27 -> [u8_GetCAAS_VMC_Req_A]  "<u8_GetCAAS_VMC_Req_A>"
  R_BTPMS_APS_outputs_BTPMS_APS_outputs_read/1 -> Bus Selector/1
